simulink model "SVPWM"  (R2023a)
settings: Solver=FixedStepAuto  StartTime=0.0  StopTime=0.05  FixedStep=1e-5  RelTol=1e-3
libraries: spsIGBTDiodeLib x6, spsSeriesRLCBranchLib x6, spsDCVoltageSourceLib x1, simulink x1
settings Model: Creator=xuluyu  LastModifiedBy=xuluyu

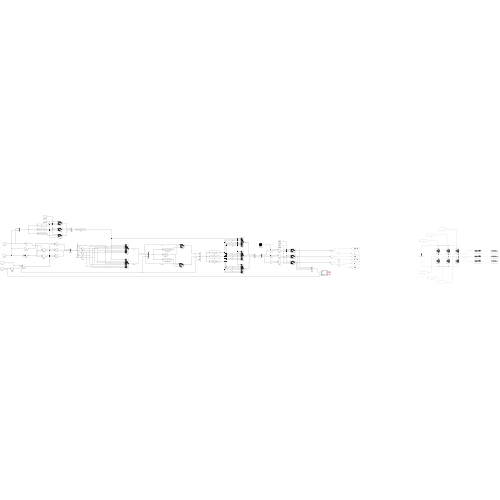
[thumbnail: Simulink's stored preview of the top-level diagram]
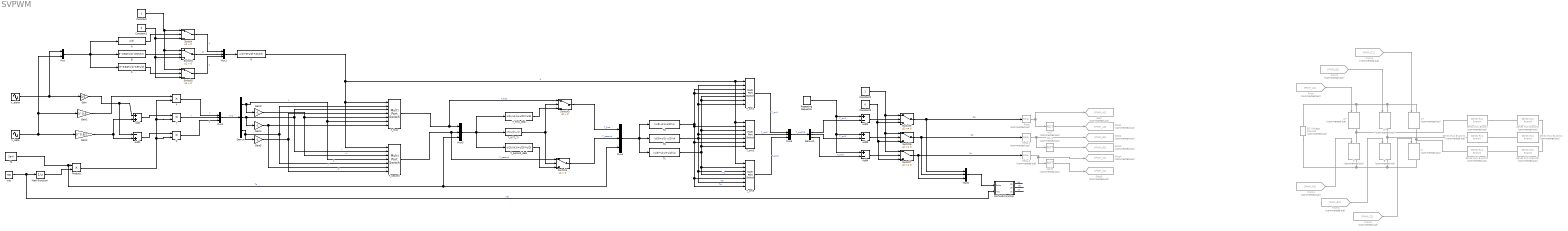
== system SVPWM ==
  A : Fcn  Expr=u(2)
  A+ : spsIGBTDiodeLib/IGBT//Diode  Commented=on  Ron=1e-3  Rs=1e5  Cs=inf  Measurements=on
  A- : spsIGBTDiodeLib/IGBT//Diode  Commented=on  Ron=1e-3  Rs=1e5  Cs=inf  Measurements=on
  Add : Sum
  Add1 : Sum  Inputs=-+
  Add2 : Sum  Inputs=+-
  Add3 : Sum  Inputs=+-
  Add4 : Sum  Inputs=+-
  B : Fcn  Expr=3^0.5/2*u(1)-0.5*u(2)
  B+ : spsIGBTDiodeLib/IGBT//Diode  Commented=on  Ron=1e-3  Rs=1e5  Cs=inf  Measurements=on
  B- : spsIGBTDiodeLib/IGBT//Diode  Commented=on  Ron=1e-3  Rs=1e5  Cs=inf  Measurements=on
  C : Fcn  Expr=-3^0.5/2*u(1)-0.5*u(2)
  C+ : spsIGBTDiodeLib/IGBT//Diode  Commented=on  Ron=1e-3  Rs=1e5  Cs=inf  Measurements=on
  C- : spsIGBTDiodeLib/IGBT//Diode  Commented=on  Ron=1e-3  Rs=1e5  Cs=inf  Measurements=on
  Constant : Constant
  Constant1 : Constant  Value=0
  Constant2 : Constant
  Constant3 : Constant  Value=0
  DC Voltage Source1 : spsDCVoltageSourceLib/DC Voltage Source  Commented=on  Amplitude=700  Measurements=None
  Demux : Demux  Outputs=3
  Demux1 : Demux  Outputs=3
  From : From  Commented=on  GotoTag=PWM_A1
  From1 : From  Commented=on  GotoTag=PWM_A2
  From2 : From  Commented=on  GotoTag=PWM_B1
  From3 : From  Commented=on  GotoTag=PWM_B2
  From4 : From  Commented=on  GotoTag=PWM_C1
  From5 : From  Commented=on  GotoTag=PWM_C2
  Gain : Gain  Gain=3/2
  Gain1 : Gain  Gain=3^0.5
  Gain2 : Gain  Gain=3^0.5/2
  Gain3 : Gain  Gain=-1
  Gain4 : Gain  Gain=-1
  Gain5 : Gain  Gain=-1
  Goto : Goto  Commented=on  GotoTag=PWM_A1
  Goto1 : Goto  Commented=on  GotoTag=PWM_A2
  Goto2 : Goto  Commented=on  GotoTag=PWM_B1
  Goto3 : Goto  Commented=on  GotoTag=PWM_B2
  Goto4 : Goto  Commented=on  GotoTag=PWM_C1
  Goto5 : Goto  Commented=on  GotoTag=PWM_C2
  MATLAB Function : MATLAB Function  TreatAsAtomicUnit=on
  Math Function : Math  Operator=reciprocal
  Mux : Mux  Inputs=2
  Mux{1..6} (6 alike) : Mux  Inputs=3
  N : Fcn  Expr=u(1)+2*u(2)+4*u(3)
  NOT : Logic  Commented=on  Operator=NOT  IconShape=distinctive  AllPortsSameDT=off  OutDataTypeStr=boolean
  NOT1 : Logic  Commented=on  Operator=NOT  IconShape=distinctive  AllPortsSameDT=off  OutDataTypeStr=boolean
  NOT2 : Logic  Commented=on  Operator=NOT  IconShape=distinctive  AllPortsSameDT=off  OutDataTypeStr=boolean
  Product : Product
  Relay : Relay  Commented=on
  Relay1 : Relay  Commented=on
  Relay2 : Relay  Commented=on
  Repeating Sequence : simulink/Sources/Repeating Sequence  rep_seq_t=[0 1e-4 2e-4]  rep_seq_y=[0 1e-4 0]
  Series RLC Branch : spsSeriesRLCBranchLib/Series RLC Branch  Commented=on  LConnTagsString=__new0  RConnTagsString=__new0  BranchType=RL  Resistance=0.5  Inductance=5e-3  SetiL0=off  InitialCurrent=0  Capacitance=1e-6  Setx0=off  InitialVoltage=0  Measurements=None
  Series RLC Branch1 : spsSeriesRLCBranchLib/Series RLC Branch  Commented=on  LConnTagsString=__new0  RConnTagsString=__new0  BranchType=RL  Resistance=0.5  Inductance=5e-3  SetiL0=off  InitialCurrent=0  Capacitance=1e-6  Setx0=off  InitialVoltage=0  Measurements=None
  Series RLC Branch2 : spsSeriesRLCBranchLib/Series RLC Branch  Commented=on  LConnTagsString=__new0  RConnTagsString=__new0  BranchType=RL  Resistance=0.5  Inductance=5e-3  SetiL0=off  InitialCurrent=0  Capacitance=1e-6  Setx0=off  InitialVoltage=0  Measurements=None
  Series RLC Branch3 : spsSeriesRLCBranchLib/Series RLC Branch  Commented=on  LConnTagsString=__new0  RConnTagsString=__new0  BranchType=R  Resistance=50  Inductance=5e-3  SetiL0=off  InitialCurrent=0  Capacitance=1e-6  Setx0=off  InitialVoltage=0  Measurements=None
  Series RLC Branch4 : spsSeriesRLCBranchLib/Series RLC Branch  Commented=on  LConnTagsString=__new0  RConnTagsString=__new0  BranchType=R  Resistance=50  Inductance=5e-3  SetiL0=off  InitialCurrent=0  Capacitance=1e-6  Setx0=off  InitialVoltage=0  Measurements=None
  Series RLC Branch5 : spsSeriesRLCBranchLib/Series RLC Branch  Commented=on  LConnTagsString=__new0  RConnTagsString=__new0  BranchType=R  Resistance=50  Inductance=5e-3  SetiL0=off  InitialCurrent=0  Capacitance=1e-6  Setx0=off  InitialVoltage=0  Measurements=None
  Switch{,1..4} (5 alike) : Switch  Criteria=u2 > Threshold  SaturateOnIntegerOverflow=off  InputSameDT=off
  Switch5 : Switch  SaturateOnIntegerOverflow=off  InputSameDT=off
  Switch6 : Switch  SaturateOnIntegerOverflow=off  InputSameDT=off
  Switch7 : Switch  SaturateOnIntegerOverflow=off  InputSameDT=off
  T_0((T_7) : Fcn  Expr=u(3)-u(2)-u(1)
  T_cm1 : MultiPortSwitch  Inputs=6  SaturateOnIntegerOverflow=off  InputSameDT=off
  T_cm2 : MultiPortSwitch  Inputs=6  SaturateOnIntegerOverflow=off  InputSameDT=off
  T_cm3 : MultiPortSwitch  Inputs=6  SaturateOnIntegerOverflow=off  InputSameDT=off
  T_first : MultiPortSwitch  Inputs=6  SaturateOnIntegerOverflow=off  InputSameDT=off
  T_first_deal : Fcn  Expr=u(1)/(u(1)+u(2))*u(3)
  T_second : MultiPortSwitch  Inputs=6  SaturateOnIntegerOverflow=off  InputSameDT=off
  T_second_deal : Fcn  Expr=u(2)/(u(1)+u(2))*u(3)
  Ta : Fcn  Expr=(u(3)-u(1)-u(2))/4
  Tb : Fcn  Expr=(u(3)+u(1)-u(2))/4
  Tc : Fcn  Expr=(u(3)+u(1)+u(2))/4
  Ts : Constant  Value=2e-4
  V_alpha : Sin  Amplitude=200  Frequency=100*pi  Phase=pi/2  SampleTime=0
  V_beta : Sin  Amplitude=200  Frequency=100*pi  SampleTime=0
  Vdc : Constant  Value=700
  X : Product
  Y : Product
  Z : Product
  wires:
  V_alpha/1 -> Mux/1, Gain/1
  V_beta/1 -> Mux/2, Gain1/1, Gain2/1
  Mux/1 -> C/1, B/1, A/1
  Mux1/1 -> N/1
  Constant/1 -> Switch2/1, Switch1/1, Switch/1
  Constant1/1 -> Switch2/3, Switch1/3, Switch/3
  A/1 -> Switch/2
  B/1 -> Switch1/2
  C/1 -> Switch2/2
  Switch/1 -> Mux1/1  "A"
  Switch1/1 -> Mux1/2  "B"
  Switch2/1 -> Mux1/3  "C"
  N/1 -> T_cm3/1, T_cm2/1, T_cm1/1, T_second/1, T_first/1  "N"
  Vdc/1 -> MATLAB Function/2(Vdc), Math Function/1  "Vdc"
  Math Function/1 -> Product/2
  Ts/1 -> Mux4/3, Mux3/3, Product/1  "Ts"
  Gain1/1 -> X/1
  Product/1 -> Z/2, Y/2, X/2
  Gain/1 -> Add1/1, Add/1
  Gain2/1 -> Add1/2, Add/2
  Add/1 -> Y/1
  Add1/1 -> Z/1
  X/1 -> Mux2/1  "X"
  Y/1 -> Mux2/2  "Y"
  Z/1 -> Mux2/3  "Z"
  Mux2/1 -> Demux/1  "XYZ"
  T_first/1 -> Switch3/1, Mux3/1  "T_first"
  T_second/1 -> Switch4/1, Mux3/2  "T_second"
  Demux/1 -> T_first/6, T_second/4, Gain3/1  "X"
  Demux/2 -> T_second/2, T_first/3, Gain4/1  "Y"
  Demux/3 -> T_second/5, T_first/2, Gain5/1  "Z"
  Gain3/1 -> T_second/3, T_first/5  "-X"
  Gain4/1 -> T_second/6, T_first/7  "-Y"
  Gain5/1 -> T_second/7, T_first/4  "-Z"
  Mux3/1 -> T_second_deal/1, T_first_deal/1, T_0((T_7)/1
  T_0((T_7)/1 -> Switch4/2, Switch3/2
  T_first_deal/1 -> Switch3/3
  T_second_deal/1 -> Switch4/3
  Switch3/1 -> Mux4/1  "T_first"
  Switch4/1 -> Mux4/2  "T_second"
  Mux4/1 -> Tc/1, Ta/1, Tb/1
  Ta/1 -> T_cm1/4, T_cm1/3, T_cm3/7, T_cm3/5, T_cm2/6, T_cm2/2  "Ta"
  Tb/1 -> T_cm2/5, T_cm2/4, T_cm1/7, T_cm1/2, T_cm3/6, T_cm3/3  "Tb"
  Tc/1 -> T_cm1/6, T_cm1/5, T_cm2/3, T_cm2/7, T_cm3/4, T_cm3/2  "Tc"
  T_cm1/1 -> Mux5/1  "T_cm1"
  T_cm2/1 -> Mux5/2  "T_cm2"
  T_cm3/1 -> Mux5/3  "T_cm3"
  Mux5/1 -> Demux1/1  "T_mc123"
  Repeating Sequence/1 -> Add4/1, Add3/1, Add2/1
  Demux1/1 -> Add2/2  "T_cm1"
  Demux1/2 -> Add3/2  "T_cm2"
  Demux1/3 -> Add4/2  "T_cm3"
  Add2/1 -> Switch5/2
  Add3/1 -> Switch6/2
  Add4/1 -> Switch7/2
  Constant2/1 -> Switch7/1, Switch6/1, Switch5/1
  Constant3/1 -> Switch7/3, Switch6/3, Switch5/3
  Switch5/1 -> Mux6/1, Relay/1  "Sa"
  Switch6/1 -> Mux6/2, Relay1/1  "Sb"
  Switch7/1 -> Mux6/3, Relay2/1  "Sc"
  Relay/1 -> Goto/1, NOT/1
  Relay1/1 -> Goto2/1, NOT1/1
  Relay2/1 -> Goto4/1, NOT2/1
  NOT/1 -> Goto1/1
  NOT1/1 -> Goto3/1
  NOT2/1 -> Goto5/1
  From/1 -> A+/1
  From1/1 -> A-/1
  From2/1 -> B+/1
  From3/1 -> B-/1
  From4/1 -> C+/1
  From5/1 -> C-/1
  Mux6/1 -> MATLAB Function/1(Sabc)
  MATLAB Function/1(Ua) -> ?  "Ua"
  MATLAB Function/2(Ub) -> ?  "Ub"
  MATLAB Function/3(Uc) -> ?  "Uc"
  connections:
  DC Voltage Source1/RConn1 -- A+/LConn1 -- B+/LConn1 -- C+/LConn1
  DC Voltage Source1/LConn1 -- A-/RConn1 -- B-/RConn1 -- C-/RConn1
  A+/RConn1 -- Series RLC Branch/LConn1 -- A-/LConn1
  B+/RConn1 -- Series RLC Branch1/LConn1 -- B-/LConn1
  C+/RConn1 -- Series RLC Branch2/LConn1 -- C-/LConn1
  Series RLC Branch5/LConn1 -- Series RLC Branch2/RConn1
  Series RLC Branch/RConn1 -- Series RLC Branch3/LConn1
  Series RLC Branch1/RConn1 -- Series RLC Branch4/LConn1
  Series RLC Branch3/RConn1 -- Series RLC Branch4/RConn1 -- Series RLC Branch5/RConn1

== matlab function SVPWM/MATLAB Function ==
  data: Sabc input; Ua output; Vdc input; Ub output; Uc output
function [Ua,Ub,Uc] = fcn(Sabc,Vdc)
    Ua = Vdc/3*(2*Sabc(1)-1*Sabc(2)-1*Sabc(3));
    Ub = Vdc/3*(-1*Sabc(1)+2*Sabc(2)-1*Sabc(3));
    Uc = Vdc/3*(-1*Sabc(1)-1*Sabc(2)+2*Sabc(3));
end
